simulink model "t2"  (R2019b)
settings: Solver=VariableStepAuto  StartTime=0.0  StopTime=5  RelTol=1e-3
libraries: powerlib x21, powerlib_meascontrol x5
settings Model: Creator=96547  LastModifiedBy=96547
settings DataIOCC: ReturnWorkspaceOutputs=off

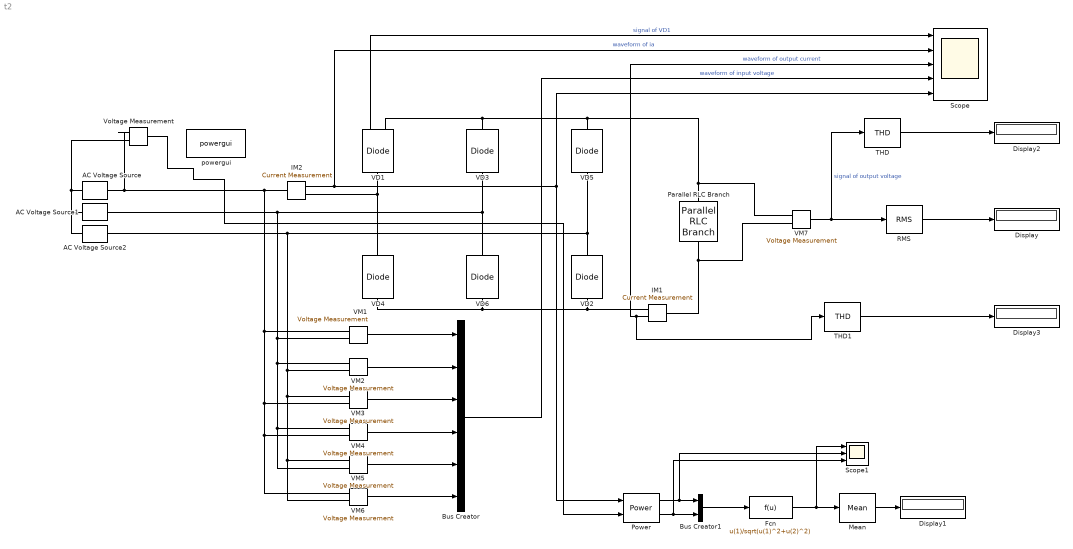
== system t2 ==
  AC Voltage Source : powerlib/Electrical Sources/AC Voltage Source  Amplitude=220*sqrt(2)  Phase=0  Frequency=50  SampleTime=0  Measurements=None  BusType=swing  Pref=10e3  Qref=0  Qmin=-inf  Qmax=+inf
      settings: SourceProductName=Simscape Electrical
  AC Voltage Source1 : powerlib/Electrical Sources/AC Voltage Source  Amplitude=220*sqrt(2)  Phase=-120  Frequency=50  SampleTime=0  Measurements=None  BusType=swing  Pref=10e3  Qref=0  Qmin=-inf  Qmax=+inf
      settings: SourceProductName=Simscape Electrical
  AC Voltage Source2 : powerlib/Electrical Sources/AC Voltage Source  Amplitude=220*sqrt(2)  Phase=-240  Frequency=50  SampleTime=0  Measurements=None  BusType=swing  Pref=10e3  Qref=0  Qmin=-inf  Qmax=+inf
      settings: SourceProductName=Simscape Electrical
  Bus Creator : BusCreator  Inputs=6
  Bus Creator1 : BusCreator  Inputs=2
  Display{,1..3} (4 alike) : Display
  Fcn : Fcn  Expr=u(1)/sqrt(u(1)^2+u(2)^2)
  IM1 : powerlib/Measurements/Current Measurement  PhasorSimulation=off  OutputType=Complex  PSBequivalent=0
      settings: SourceProductName=Simscape Electrical
  IM2 : powerlib/Measurements/Current Measurement  PhasorSimulation=off  OutputType=Complex  PSBequivalent=0
      settings: SourceProductName=Simscape Electrical
  Mean : powerlib_meascontrol/Measurements/Mean  Freq=60  Vinit=0  Ts=0
      settings: SourceProductName=Simscape Electrical
  Parallel RLC Branch : powerlib/Elements/Parallel RLC Branch  LConnTagsString=a  RConnTagsString=__new0  BranchType=RC  Resistance=10000  Inductance=1e-3  SetiL0=off  InitialCurrent=0  Capacitance=5.5e-3  Setx0=off  InitialVoltage=0  Measurements=None
      settings: SourceProductName=Simscape Electrical
  Power : powerlib_meascontrol/Measurements/Power  Freq=60  Vinit=[1, 0]  Iinit=[1, 0]  Ts=0
      settings: SourceProductName=Simscape Electrical
  RMS : powerlib_meascontrol/Measurements/RMS  TrueRMS=on  Freq=60  RMSInit=120  Ts=0
      settings: SourceProductName=Simscape Electrical
  Scope : Scope  NumInputPorts=5
  Scope1 : Scope  NumInputPorts=3
  THD : powerlib_meascontrol/Measurements/THD  Freq=60  Ts=0
      settings: SourceProductName=Simscape Electrical
  THD1 : powerlib_meascontrol/Measurements/THD  Freq=60  Ts=0
      settings: SourceProductName=Simscape Electrical
  VD1 : powerlib/Power Electronics/Diode  Ron=0.001  Lon=0  Vf=0.8  IC=0  UseSnubber=0  Rs=500  Cs=250e-9  Measurements=on
      settings: SourceProductName=Simscape Electrical
  VD{2..6} (5 alike) : powerlib/Power Electronics/Diode  Ron=0.001  Lon=0  Vf=0.8  IC=0  UseSnubber=0  Rs=500  Cs=250e-9  Measurements=off
      settings: SourceProductName=Simscape Electrical
  VM{1..7} (7 alike) : powerlib/Measurements/Voltage Measurement  PhasorSimulation=off  OutputType=Complex  PSBequivalent=0
      settings: SourceProductName=Simscape Electrical
  Voltage Measurement : powerlib/Measurements/Voltage Measurement  PhasorSimulation=off  OutputType=Complex  PSBequivalent=0
      settings: SourceProductName=Simscape Electrical
  powergui : powerlib/powergui  Priority=1  SimulationMode=Continuous  SampleTime=50e-6  frequency=60  Iterations=50  frequencyindice=50  Pbase=100e6  ErrMax=1e-4  UnitsV=kV  UnitsW=MW  buscounter=0  FunctionMessages=off  echomessages=off  EnableUseOfTLC=off  CurrentSourceSwitches=off  DisableSnubberDevices=off  DisableRonSwitches=off  DisableVfSwitches=off  DisplayEquations=off  AutomaticDiscreteSolvers=off  SolverType=Tustin/Backward Euler (TBE)  Interpol=off  ExternalGateDelay=off  methode=off  Ts=100  x0status=blocks  SPID=on  SwTol=0  HookPort=off  NonlinearTolerance=1e-4  nMaxIteration=100  ContinueOnMaxIteration=off  RestoreLinks=warning  ResistiveCurrentMeasurement=off  Frange=[0:2:500]  Ylog=off  Xlog=on  ShowGrid=off  save=off  variable=ZData  structure=v1  ZoomFFT=off  StartTime=0.01  cycles=1  DisplayStyle=1  fundamental=50  FreqAxis=off  MaxFrequency=1000  frequencyindicesteady=1  RmsSteady=1  display=off
      settings: SourceProductName=Simscape Electrical
  wires:
  VM1/1 -> Bus Creator/1
  VM2/1 -> Bus Creator/2
  VM3/1 -> Bus Creator/3
  VM4/1 -> Bus Creator/4
  VM5/1 -> Bus Creator/5
  VM6/1 -> Bus Creator/6
  VM7/1 -> RMS/1, THD/1  "signal of output voltage"
  IM1/1 -> THD1/1, Scope/3  "waveform of output current"
  Bus Creator/1 -> Scope/4  "waveform of input voltage"
  VD1/1 -> Scope/1  "signal of VD1"
  IM2/1 -> Scope/2, Power/1, Scope/5  "waveform of ia"
  RMS/1 -> Display/1
  THD/1 -> Display2/1
  THD1/1 -> Display3/1
  Voltage Measurement/1 -> Power/2
  Power/1 -> Scope1/2, Bus Creator1/1
  Power/2 -> Scope1/3, Bus Creator1/2
  Bus Creator1/1 -> Fcn/1
  Fcn/1 -> Mean/1, Scope1/1
  Mean/1 -> Display1/1
  connections:
  AC Voltage Source/RConn1 -- VM6/LConn1 -- VM4/LConn2 -- VM3/LConn2 -- VM1/LConn1 -- IM2/LConn1 -- Voltage Measurement/LConn1
  VD3/LConn1 -- AC Voltage Source1/RConn1 -- VM5/LConn2 -- VM4/LConn1 -- VM2/LConn1 -- VM1/LConn2 -- VD6/RConn1
  VD5/LConn1 -- AC Voltage Source2/RConn1 -- VM6/LConn2 -- VM5/LConn1 -- VM3/LConn1 -- VM2/LConn2 -- VD2/RConn1
  Parallel RLC Branch/LConn1 -- VM7/LConn1 -- VD1/RConn1 -- VD3/RConn1 -- VD5/RConn1
  VD4/LConn1 -- IM1/RConn1 -- VD2/LConn1 -- VD6/LConn1
  AC Voltage Source/LConn1 -- Voltage Measurement/LConn2 -- AC Voltage Source2/LConn1 -- AC Voltage Source1/LConn1
  VM7/LConn2 -- Parallel RLC Branch/RConn1 -- IM1/LConn1
  VD1/LConn1 -- IM2/RConn1 -- VD4/RConn1
